simulink model "mainmodel"  (R2020a)
settings: Solver=VariableStepAuto  StartTime=0.0  StopTime=10.0  RelTol=1e-3
PreLoadFcn:
  | R = 10;
  | C = 10e-6;
settings Model: Creator=Bhanu  LastModifiedBy=Bhanu

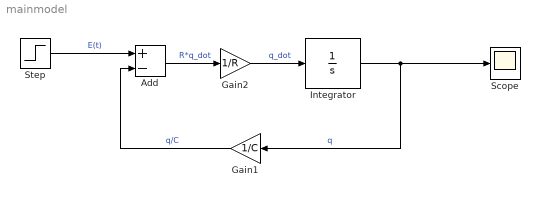
== system mainmodel ==
  Add : Sum  Inputs=+-
  Gain1 : Gain  Gain=1/C
  Gain2 : Gain  Gain=1/R
  Integrator : Integrator
  Scope : Scope
  Step : Step  SampleTime=0
  wires:
  Integrator/1 -> Gain1/1, Scope/1  "q"
  Add/1 -> Gain2/1  "R*q_dot"
  Gain1/1 -> Add/2  "q/C"
  Gain2/1 -> Integrator/1  "q_dot"
  Step/1 -> Add/1  "E(t)"
